simulink model "APP_DD2"  (R2018a)
settings: configuration reference "cs_ert" (kept outside this file)
settings Model: DataDictionary=APP_DD2.sldd  Creator=zhoutinglin  LastModifiedBy=zhoutinglin

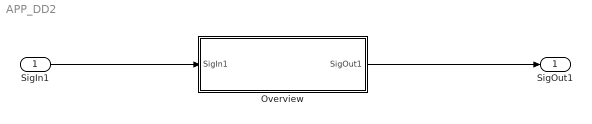
== system APP_DD2 ==
  SigIn1 : Inport  OutDataTypeStr=uint8
  Overview : Subsystem
  SigOut1 : Outport
  wires:
  Overview/1(SigOut1) -> SigOut1/1
  SigIn1/1 -> Overview/1(SigIn1)

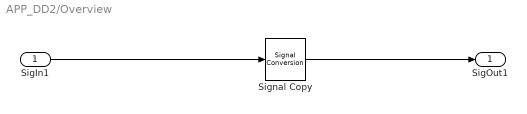
== system APP_DD2/Overview ==
  SigIn1 : Inport
  Signal Copy : SignalConversion  OverrideOpt=off
  SigOut1 : Outport
  wires:
  SigIn1/1 -> Signal Copy/1
  Signal Copy/1 -> SigOut1/1
